simulink model "s01_unicycle"  (R2020a)
settings: Solver=VariableStepAuto  StartTime=0.0  StopTime=20  FixedStep=0.001
InitFcn:
  | clc, close all
  | 
  | run('./s00_config.m')
  | 
  | load('./parameters/ut_obj')
  | load('./parameters/yt_obj')
  | load('./parameters/Kp')
  | load('./parameters/Kr')
  | load('./parameters/Mp')
  | load('./parameters/Mr')
  | 
  | iterSeed = randi(500);
model workspace (MAT data in the model file):
  M : object (value not decoded)
  M_nonlin : object (value not decoded)
  M_tmp : object (value not decoded)
  RHS : object (value not decoded)
  RHS_nonlin : object (value not decoded)
  RHS_tmp : object (value not decoded)
  Tp : object (value not decoded)
  Tp_var = 0
  Tw : object (value not decoded)
  Tw_var = 0
  op_trim3 : handle (value not decoded)
  q1 : object (value not decoded)
  q1_d : object (value not decoded)
  q2 : object (value not decoded)
  q2_d : object (value not decoded)
  q3 : object (value not decoded)
  q3_d : object (value not decoded)
  q4 : object (value not decoded)
  q4_d : object (value not decoded)
  q5 : object (value not decoded)
  q5_d : object (value not decoded)
  z = [0 0 0 0 0 0 0 0 0 0 0 0 ... (100 elements, 10x10)]
values from neighbouring files (symbols this model uses):
  b_disc = 0.01    [s00_config.m]
  Bp = [B_p1 B_p2 B_p3 B_p4]    [s00_config.m]    (also in s00_designLQR.m = double([0; b2; 0; b4]))
  flag_AddPitchBias = 0    [s00_config.m]
  flag_AddRollBias = 0    [s00_config.m]
  flag_UseAccNoise = 1    [s00_config.m]
  flag_useControlDelay = 0    [s00_config.m]
  flag_UseGyroNoise = 1    [s00_config.m]
  flag_UsePitchEst = 1    [s00_config.m]
  flag_UsePivotAcc = 1    [s00_config.m]
  flag_UseRateEst = 1    [s00_config.m]
  flag_UseRollEst = 1    [s00_config.m]
  flag_UseYawEst = 1    [s00_config.m]
  Icx = 0.001746    [s00_config.m]
  Icy = 0.00181    [s00_config.m]
  Icz = 0.001585    [s00_config.m]
  Iwx = 0.000259    [s00_config.m]
  Iwy = 0.000503    [s00_config.m]
  Iwz = 0.000259    [s00_config.m]
  Lc = 0.055    [s00_config.m]
  Lcp = 0.055    [s00_config.m]
  mean_IMUgyro = -0.0065    [s00_config.m]
  pitch_bias = deg2rad(1)    [s00_config.m]
  q1_0 = -deg2rad(36)    [s00_config.m]
  q2_0 = deg2rad(0)    [s00_config.m]
  r = Rw - 0.01    (= 0.043)    [s00_config.m]
  roll_bias = deg2rad(1)    [s00_config.m]
  Rw = 0.053    [s00_config.m]
  stall_torque = 1.6    [s00_config.m]
  Ts = 1/100    (= 0.01)    [s00_config.m]
  variance_IMUacc = 0.0049    [s00_config.m]
  variance_IMUgyro = 6.3956e-04    (= 0.00063956)    [s00_config.m]
  X = (P.')/(P*P.')    [s00_config.m]
  Xp = X(:,1)    [s00_config.m]
undefined symbols (not defined in the file or in its folder): DiscIntNeverNeededParam, sigbuilder_block, Y, Z
libraries: sm_lib x59, aerolibconvert2 x11, nesl_utility x8, eeGeneralControl x2, simulink x1, SignalEditorBlockLib x1
(part 2 of 2)

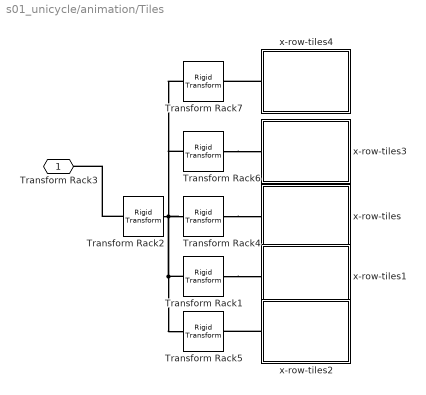
== system s01_unicycle/animation/Tiles ==
  Transform Rack1 : sm_lib/Frames and Transforms/Rigid Transform  TranslationMethod=StandardAxis  TranslationStandardOffset=0.25  TranslationLengthUnit=m  TranslationStandardAxis=-Y  TranslationCartesianOffset=[0 0 0]  TranslationROffset=0  TranslationROffsetUnits=m  TranslationZOffset=0  TranslationZOffsetUnits=m  TranslationThetaOffset=0  TranslationThetaOffsetUnits=deg  RotationMethod=None  RotationAngleUnits=deg  RotationStandardAxis=-X  RotationAngle=90  RotationArbitraryAxis=[0 0 1]  FollAlignAxisA=+X  BaseAlignAxisA=+Y  FollAlignAxisB=+Y  BaseAlignAxisB=+Z  RotationSequenceAxes=FollowerAxes  RotationSequence=XYX  RotationSequenceAngles=[0 0 0]  RotationSequenceAnglesUnits=deg  RotationMatrix=[1 0 0; 0 1 0; 0 0 1]
  Transform Rack2 : sm_lib/Frames and Transforms/Rigid Transform  TranslationMethod=StandardAxis  TranslationStandardOffset=0.001  TranslationLengthUnit=m  TranslationStandardAxis=+Z  TranslationCartesianOffset=[0 0 0]  TranslationROffset=0  TranslationROffsetUnits=m  TranslationZOffset=0  TranslationZOffsetUnits=m  TranslationThetaOffset=0  TranslationThetaOffsetUnits=deg  RotationMethod=None  RotationAngleUnits=deg  RotationStandardAxis=-X  RotationAngle=90  RotationArbitraryAxis=[0 0 1]  FollAlignAxisA=+X  BaseAlignAxisA=+Y  FollAlignAxisB=+Y  BaseAlignAxisB=+Z  RotationSequenceAxes=FollowerAxes  RotationSequence=XYX  RotationSequenceAngles=[0 0 0]  RotationSequenceAnglesUnits=deg  RotationMatrix=[1 0 0; 0 1 0; 0 0 1]
  Transform Rack4 : sm_lib/Frames and Transforms/Rigid Transform  TranslationMethod=StandardAxis  TranslationStandardOffset=0  TranslationLengthUnit=m  TranslationStandardAxis=-Y  TranslationCartesianOffset=[0 0 0]  TranslationROffset=0  TranslationROffsetUnits=m  TranslationZOffset=0  TranslationZOffsetUnits=m  TranslationThetaOffset=0  TranslationThetaOffsetUnits=deg  RotationMethod=None  RotationAngleUnits=deg  RotationStandardAxis=-X  RotationAngle=90  RotationArbitraryAxis=[0 0 1]  FollAlignAxisA=+X  BaseAlignAxisA=+Y  FollAlignAxisB=+Y  BaseAlignAxisB=+Z  RotationSequenceAxes=FollowerAxes  RotationSequence=XYX  RotationSequenceAngles=[0 0 0]  RotationSequenceAnglesUnits=deg  RotationMatrix=[1 0 0; 0 1 0; 0 0 1]
  Transform Rack5 : sm_lib/Frames and Transforms/Rigid Transform  TranslationMethod=StandardAxis  TranslationStandardOffset=0.25  TranslationLengthUnit=m  TranslationStandardAxis=+Y  TranslationCartesianOffset=[0 0 0]  TranslationROffset=0  TranslationROffsetUnits=m  TranslationZOffset=0  TranslationZOffsetUnits=m  TranslationThetaOffset=0  TranslationThetaOffsetUnits=deg  RotationMethod=None  RotationAngleUnits=deg  RotationStandardAxis=-X  RotationAngle=90  RotationArbitraryAxis=[0 0 1]  FollAlignAxisA=+X  BaseAlignAxisA=+Y  FollAlignAxisB=+Y  BaseAlignAxisB=+Z  RotationSequenceAxes=FollowerAxes  RotationSequence=XYX  RotationSequenceAngles=[0 0 0]  RotationSequenceAnglesUnits=deg  RotationMatrix=[1 0 0; 0 1 0; 0 0 1]
  Transform Rack6 : sm_lib/Frames and Transforms/Rigid Transform  TranslationMethod=StandardAxis  TranslationStandardOffset=0.5  TranslationLengthUnit=m  TranslationStandardAxis=-Y  TranslationCartesianOffset=[0 0 0]  TranslationROffset=0  TranslationROffsetUnits=m  TranslationZOffset=0  TranslationZOffsetUnits=m  TranslationThetaOffset=0  TranslationThetaOffsetUnits=deg  RotationMethod=None  RotationAngleUnits=deg  RotationStandardAxis=-X  RotationAngle=90  RotationArbitraryAxis=[0 0 1]  FollAlignAxisA=+X  BaseAlignAxisA=+Y  FollAlignAxisB=+Y  BaseAlignAxisB=+Z  RotationSequenceAxes=FollowerAxes  RotationSequence=XYX  RotationSequenceAngles=[0 0 0]  RotationSequenceAnglesUnits=deg  RotationMatrix=[1 0 0; 0 1 0; 0 0 1]
  Transform Rack7 : sm_lib/Frames and Transforms/Rigid Transform  TranslationMethod=StandardAxis  TranslationStandardOffset=0.5  TranslationLengthUnit=m  TranslationStandardAxis=+Y  TranslationCartesianOffset=[0 0 0]  TranslationROffset=0  TranslationROffsetUnits=m  TranslationZOffset=0  TranslationZOffsetUnits=m  TranslationThetaOffset=0  TranslationThetaOffsetUnits=deg  RotationMethod=None  RotationAngleUnits=deg  RotationStandardAxis=-X  RotationAngle=90  RotationArbitraryAxis=[0 0 1]  FollAlignAxisA=+X  BaseAlignAxisA=+Y  FollAlignAxisB=+Y  BaseAlignAxisB=+Z  RotationSequenceAxes=FollowerAxes  RotationSequence=XYX  RotationSequenceAngles=[0 0 0]  RotationSequenceAnglesUnits=deg  RotationMatrix=[1 0 0; 0 1 0; 0 0 1]
  x-row-tiles : Subsystem
  x-row-tiles1 : Subsystem
  x-row-tiles2 : Subsystem
  x-row-tiles3 : Subsystem
  x-row-tiles4 : Subsystem
  Transform Rack3 : PMIOPort  Side=Left
  connections:
  Transform Rack1/LConn1 -- Transform Rack7/LConn1 -- Transform Rack6/LConn1 -- Transform Rack4/LConn1 -- Transform Rack2/RConn1 -- Transform Rack5/LConn1
  x-row-tiles4/LConn1 -- Transform Rack7/RConn1
  x-row-tiles2/LConn1 -- Transform Rack5/RConn1
  Transform Rack4/RConn1 -- x-row-tiles/LConn1
  Transform Rack1/RConn1 -- x-row-tiles1/LConn1
  Transform Rack2/LConn1 -- Transform Rack3/RConn1
  Transform Rack6/RConn1 -- x-row-tiles3/LConn1

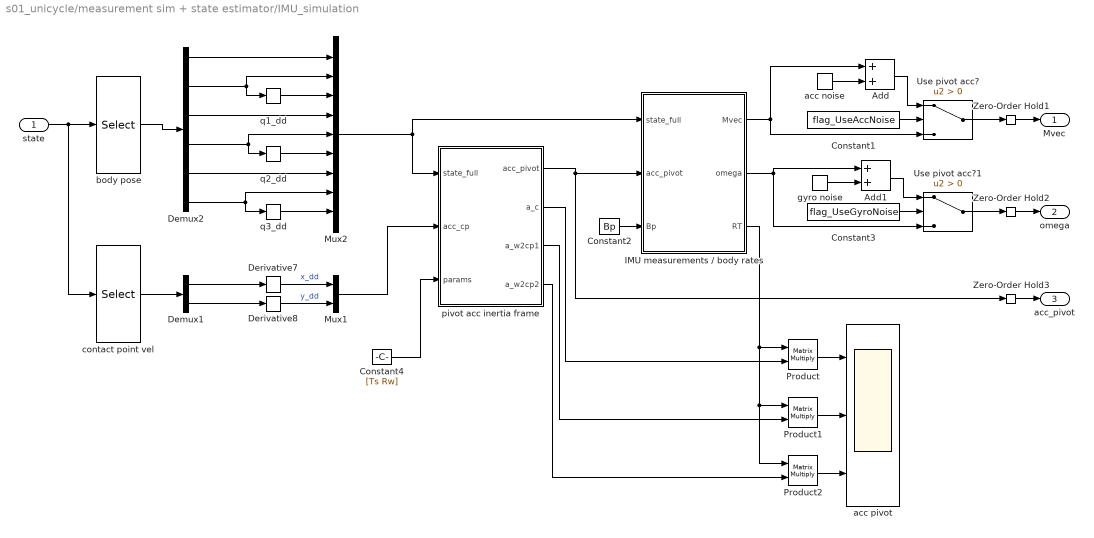
== system s01_unicycle/measurement sim + state estimator/IMU_simulation ==
  state : Inport
  Add : Sum
  Add1 : Sum
  Constant1 : Constant  Value=flag_UseAccNoise
  Constant2 : Constant  Value=Bp
  Constant3 : Constant  Value=flag_UseGyroNoise
  Constant4 : Constant  Value=[Ts Rw]
  Demux1 : Demux  Outputs=2
  Demux2 : Demux  Outputs=6
  Derivative7 : Derivative  CoefficientInTFapproximation=0.00001
  Derivative8 : Derivative  CoefficientInTFapproximation=0.00001
  IMU measurements / body rates : MATLAB Function  TreatAsAtomicUnit=on
  Mux1 : Mux  Inputs=2
  Mux2 : Mux  Inputs=9
  Product : Product  Multiplication=Matrix(*)
  Product1 : Product  Multiplication=Matrix(*)
  Product2 : Product  Multiplication=Matrix(*)
  Use pivot acc? : Switch  Criteria=u2 > Threshold
  Use pivot acc?1 : Switch  Criteria=u2 > Threshold
  Zero-Order Hold1 : ZeroOrderHold  SampleTime=Ts
  Zero-Order Hold2 : ZeroOrderHold  SampleTime=Ts
  Zero-Order Hold3 : ZeroOrderHold  SampleTime=Ts
  acc noise : RandomNumber  Mean=zeros(1,12)  Variance=variance_IMUacc*ones(1,12)  Seed=1:12  SampleTime=Ts
  acc pivot : Scope  NumInputPorts=3
  body pose : Selector  InputPortWidth=14  IndexOptions=Index vector (dialog)  Indices=[1 2 3 4 5 6]  OutputSizes=1
  contact point vel : Selector  InputPortWidth=14  IndexOptions=Index vector (dialog)  Indices=[13, 14]  OutputSizes=1
  gyro noise : RandomNumber  Mean=mean_IMUgyro*[1 1 1]  Variance=(variance_IMUgyro)*[1 1 1]  Seed=[iterSeed+10 iterSeed+11 iterSeed+12]  SampleTime=Ts
  pivot acc inertia frame : MATLAB Function  TreatAsAtomicUnit=on
  q1_dd : Derivative  CoefficientInTFapproximation=0.0000001
  q2_dd : Derivative  CoefficientInTFapproximation=0.000001
  q3_dd : Derivative  CoefficientInTFapproximation=0.000001
  Mvec : Outport
  omega : Outport  Port=2
  acc_pivot : Outport  Port=3
  wires:
  Demux2/2 -> Mux2/2, q1_dd/1
  Mux2/1 -> IMU measurements / body rates/1(state_full), pivot acc inertia frame/1(state_full)
  state/1 -> contact point vel/1, body pose/1
  Demux2/6 -> Mux2/8, q3_dd/1
  Demux1/1 -> Derivative7/1
  gyro noise/1 -> Add1/2
  IMU measurements / body rates/1(Mvec) -> Use pivot acc?/3, Add/1
  Constant2/1 -> IMU measurements / body rates/3(Bp)
  Demux2/4 -> Mux2/5, q2_dd/1
  IMU measurements / body rates/2(omega) -> Use pivot acc?1/3, Add1/1
  q2_dd/1 -> Mux2/6
  q1_dd/1 -> Mux2/3
  contact point vel/1 -> Demux1/1
  Derivative8/1 -> Mux1/2  "y_dd"
  Demux2/5 -> Mux2/7
  Demux2/1 -> Mux2/1
  Mux1/1 -> pivot acc inertia frame/2(acc_cp)
  pivot acc inertia frame/1(acc_pivot) -> Zero-Order Hold3/1, IMU measurements / body rates/2(acc_pivot)
  Derivative7/1 -> Mux1/1  "x_dd"
  body pose/1 -> Demux2/1
  Demux2/3 -> Mux2/4
  Demux1/2 -> Derivative8/1
  acc noise/1 -> Add/2
  q3_dd/1 -> Mux2/9
  Constant4/1 -> pivot acc inertia frame/3(params)
  Zero-Order Hold1/1 -> Mvec/1
  Zero-Order Hold2/1 -> omega/1
  Zero-Order Hold3/1 -> acc_pivot/1
  Use pivot acc?/1 -> Zero-Order Hold1/1
  Add/1 -> Use pivot acc?/1
  Constant1/1 -> Use pivot acc?/2
  Constant3/1 -> Use pivot acc?1/2
  Use pivot acc?1/1 -> Zero-Order Hold2/1
  Add1/1 -> Use pivot acc?1/1
  pivot acc inertia frame/2(a_c) -> Product/2
  pivot acc inertia frame/3(a_w2cp1) -> Product1/2
  pivot acc inertia frame/4(a_w2cp2) -> Product2/2
  IMU measurements / body rates/3(RT) -> Product2/1, Product1/1, Product/1
  Product/1 -> acc pivot/1
  Product2/1 -> acc pivot/3
  Product1/1 -> acc pivot/2

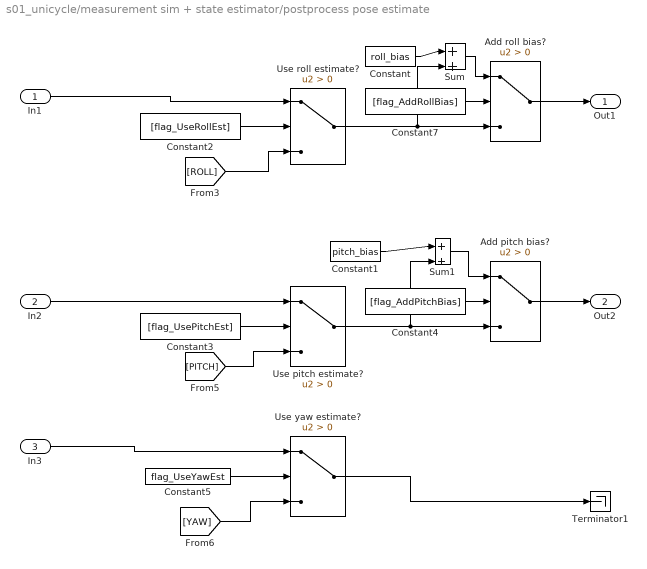
== system s01_unicycle/measurement sim + state estimator/postprocess pose estimate ==
  In1 : Inport
  In2 : Inport  Port=2
  In3 : Inport  Port=3
  Add pitch bias? : Switch  Criteria=u2 > Threshold
  Add roll bias? : Switch  Criteria=u2 > Threshold
  Constant : Constant  Value=roll_bias
  Constant1 : Constant  Value=pitch_bias
  Constant2 : Constant  Value=[flag_UseRollEst]
  Constant3 : Constant  Value=[flag_UsePitchEst]
  Constant4 : Constant  Value=[flag_AddPitchBias]
  Constant5 : Constant  Value=flag_UseYawEst
  Constant7 : Constant  Value=[flag_AddRollBias]
  Sum : Sum  Inputs=|++
  Sum1 : Sum  Inputs=|++
  Terminator1 : Terminator
  Use pitch estimate? : Switch  Criteria=u2 > Threshold
  Use roll estimate? : Switch  Criteria=u2 > Threshold
  Use yaw estimate? : Switch  Criteria=u2 > Threshold
  Out1 : Outport
  Out2 : Outport  Port=2
  wires:
  [ROLL] -> Use roll estimate?/3
  Use yaw estimate?/1 -> Terminator1/1
  Constant7/1 -> Add roll bias?/2
  Constant2/1 -> Use roll estimate?/2
  [YAW] -> Use yaw estimate?/3
  [PITCH] -> Use pitch estimate?/3
  In2/1 -> Use pitch estimate?/1
  Sum/1 -> Add roll bias?/1
  Use roll estimate?/1 -> Sum/2, Add roll bias?/3
  Constant/1 -> Sum/1
  Constant5/1 -> Use yaw estimate?/2
  Constant3/1 -> Use pitch estimate?/2
  In3/1 -> Use yaw estimate?/1
  Add roll bias?/1 -> Out1/1
  In1/1 -> Use roll estimate?/1
  Use pitch estimate?/1 -> Sum1/2, Add pitch bias?/3
  Sum1/1 -> Add pitch bias?/1
  Add pitch bias?/1 -> Out2/1
  Constant4/1 -> Add pitch bias?/2
  Constant1/1 -> Sum1/1

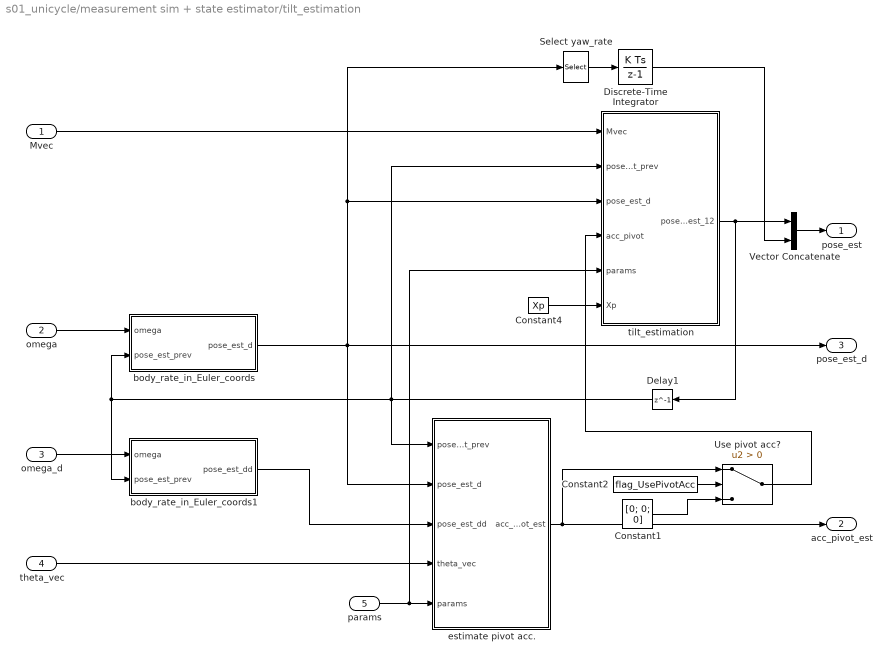
== system s01_unicycle/measurement sim + state estimator/tilt_estimation ==
  Mvec : Inport
  omega : Inport  Port=2
  omega_d : Inport  Port=3
  theta_vec : Inport  Port=4  PortDimensions=3
  params : Inport  Port=5
  Constant1 : Constant  Value="[0;  0; 0]"
  Constant2 : Constant  Value=flag_UsePivotAcc
  Constant4 : Constant  Value=Xp
  Delay1 : Delay  DelayLength=1  InitialCondition=[q1_0; q2_0]  SampleTime=Ts
  Discrete-Time Integrator : DiscreteIntegrator  SampleTime=-1  ICPrevOutput=DiscIntNeverNeededParam  ICPrevScaledInput=DiscIntNeverNeededParam
  Select yaw_rate : Selector  InputPortWidth=3  IndexOptions=Index vector (dialog)  Indices=[3]  OutputSizes=1
  Use pivot acc? : Switch  Criteria=u2 > Threshold
  Vector Concatenate : Concatenate
  body_rate_in_Euler_coords : MATLAB Function  TreatAsAtomicUnit=on
  body_rate_in_Euler_coords1 : MATLAB Function  TreatAsAtomicUnit=on
  estimate pivot acc. : MATLAB Function  TreatAsAtomicUnit=on
  tilt_estimation : MATLAB Function  TreatAsAtomicUnit=on
  pose_est : Outport
  acc_pivot_est : Outport  Port=2
  pose_est_d : Outport  Port=3
  wires:
  estimate pivot acc./1(acc_pivot_est) -> Use pivot acc?/1, acc_pivot_est/1
  Delay1/1 -> estimate pivot acc./1(pose_est_prev), body_rate_in_Euler_coords/2(pose_est_prev), body_rate_in_Euler_coords1/2(pose_est_prev), tilt_estimation/2(pose_est_prev)
  body_rate_in_Euler_coords/1(pose_est_d) -> pose_est_d/1, Select yaw_rate/1, tilt_estimation/3(pose_est_d), estimate pivot acc./2(pose_est_d)
  Select yaw_rate/1 -> Discrete-Time Integrator/1
  omega_d/1 -> body_rate_in_Euler_coords1/1(omega)
  body_rate_in_Euler_coords1/1(pose_est_dd) -> estimate pivot acc./3(pose_est_dd)
  Use pivot acc?/1 -> tilt_estimation/4(acc_pivot)
  omega/1 -> body_rate_in_Euler_coords/1(omega)
  params/1 -> tilt_estimation/5(params), estimate pivot acc./5(params)
  tilt_estimation/1(pose_est_12) -> Vector Concatenate/1, Delay1/1
  Mvec/1 -> tilt_estimation/1(Mvec)
  Vector Concatenate/1 -> pose_est/1
  Constant4/1 -> tilt_estimation/6(Xp)
  Constant1/1 -> Use pivot acc?/3
  Constant2/1 -> Use pivot acc?/2
  Discrete-Time Integrator/1 -> Vector Concatenate/2
  theta_vec/1 -> estimate pivot acc./4(theta_vec)

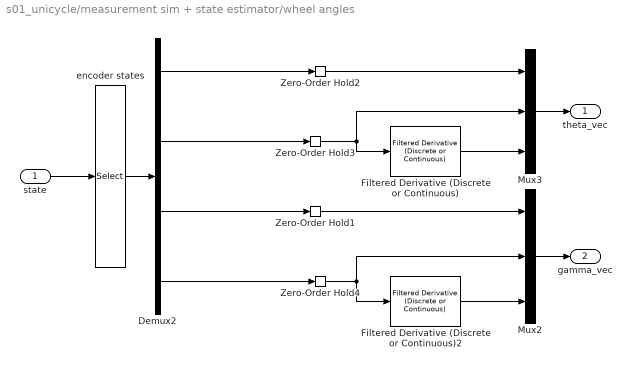
== system s01_unicycle/measurement sim + state estimator/wheel angles ==
  state : Inport
  Demux2 : Demux
  Filtered Derivative (Discrete or Continuous) : eeGeneralControl/Filtered Derivative (Discrete or Continuous)  K=1  T=0.1  B=inf  A=-inf  minRatio=10  init_option=Inherited from block input  x0=0  Ts=-1
      settings: SourceProductBaseCode=PS
  Filtered Derivative (Discrete or Continuous)2 : eeGeneralControl/Filtered Derivative (Discrete or Continuous)  K=1  T=0.1  B=inf  A=-inf  minRatio=10  init_option=Inherited from block input  x0=0  Ts=-1
      settings: SourceProductBaseCode=PS
  Mux2 : Mux  Inputs=3
  Mux3 : Mux  Inputs=3
  Zero-Order Hold{1..4} (4 alike) : ZeroOrderHold  SampleTime=Ts
  encoder states : Selector  InputPortWidth=14  IndexOptions=Index vector (dialog)  Indices=[7, 8, 9, 10]  OutputSizes=1
  theta_vec : Outport
  gamma_vec : Outport  Port=2
  wires:
  Demux2/3 -> Zero-Order Hold1/1
  encoder states/1 -> Demux2/1
  Zero-Order Hold3/1 -> Mux3/2, Filtered Derivative (Discrete or Continuous)/1
  Demux2/2 -> Zero-Order Hold3/1
  Demux2/1 -> Zero-Order Hold2/1
  state/1 -> encoder states/1
  Filtered Derivative (Discrete or Continuous)/1 -> Mux3/3
  Demux2/4 -> Zero-Order Hold4/1
  Zero-Order Hold4/1 -> Mux2/2, Filtered Derivative (Discrete or Continuous)2/1
  Filtered Derivative (Discrete or Continuous)2/1 -> Mux2/3
  Mux3/1 -> theta_vec/1
  Zero-Order Hold1/1 -> Mux2/1
  Mux2/1 -> gamma_vec/1
  Zero-Order Hold2/1 -> Mux3/1

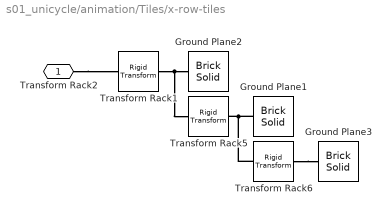
== system s01_unicycle/animation/Tiles/x-row-tiles ==
  Ground Plane1 : sm_lib/Body Elements/Brick Solid  GraphicAmbientColor=[0.15 0.15 0 1.0]  BasedOnType=Density  BrickDimensions=[0.25 0.25 0.001]  BrickDimensionUnits=m  CenterOfMass=[0 0 0]  CenterOfMassUnits=m  GraphicDiffuseColor=[1.0 1.0 1.0]  Density=100  DensityUnits=kg/(m^3)  DoExposeReferenceFrame=on  GraphicEmissiveColor=[0.0 0.0 0.0 1.0]  ExportEntireGeometry=off  SerializedFrames=<Frames/>  MarkerShape=Cube  MarkerSize=10000  GraphicType=FromGeometry  InertiaType=CalculateFromGeometry  Mass=1  MassUnits=kg  MomentsOfInertia=[1 1 1]  MomentsOfInertiaUnits=kg*m^2  GraphicOpacity=1  ProductsOfInertia=[0 0 0]  ProductsOfInertiaUnits=kg*m^2  GraphicShininess=75  GraphicSpecularColor=[0.5 0.5 0.1 1.0]  GraphicVisPropType=SimpleVisualProperties
  Ground Plane2 : sm_lib/Body Elements/Brick Solid  GraphicAmbientColor=[0.15 0.15 0 1.0]  BasedOnType=Density  BrickDimensions=[0.25 0.25 0.001]  BrickDimensionUnits=m  CenterOfMass=[0 0 0]  CenterOfMassUnits=m  GraphicDiffuseColor=[1.0 1.0 1.0]  Density=100  DensityUnits=kg/(m^3)  DoExposeReferenceFrame=on  GraphicEmissiveColor=[0.0 0.0 0.0 1.0]  ExportEntireGeometry=off  SerializedFrames=<Frames/>  MarkerShape=Cube  MarkerSize=10000  GraphicType=FromGeometry  InertiaType=CalculateFromGeometry  Mass=1  MassUnits=kg  MomentsOfInertia=[1 1 1]  MomentsOfInertiaUnits=kg*m^2  GraphicOpacity=1  ProductsOfInertia=[0 0 0]  ProductsOfInertiaUnits=kg*m^2  GraphicShininess=75  GraphicSpecularColor=[0.5 0.5 0.1 1.0]  GraphicVisPropType=SimpleVisualProperties
  Ground Plane3 : sm_lib/Body Elements/Brick Solid  GraphicAmbientColor=[0.15 0.15 0 1.0]  BasedOnType=Density  BrickDimensions=[0.25 0.25 0.001]  BrickDimensionUnits=m  CenterOfMass=[0 0 0]  CenterOfMassUnits=m  GraphicDiffuseColor=[1.0 1.0 1.0]  Density=100  DensityUnits=kg/(m^3)  DoExposeReferenceFrame=on  GraphicEmissiveColor=[0.0 0.0 0.0 1.0]  ExportEntireGeometry=off  SerializedFrames=<Frames/>  MarkerShape=Cube  MarkerSize=10000  GraphicType=FromGeometry  InertiaType=CalculateFromGeometry  Mass=1  MassUnits=kg  MomentsOfInertia=[1 1 1]  MomentsOfInertiaUnits=kg*m^2  GraphicOpacity=1  ProductsOfInertia=[0 0 0]  ProductsOfInertiaUnits=kg*m^2  GraphicShininess=75  GraphicSpecularColor=[0.5 0.5 0.1 1.0]  GraphicVisPropType=SimpleVisualProperties
  Transform Rack1 : sm_lib/Frames and Transforms/Rigid Transform  TranslationMethod=StandardAxis  TranslationStandardOffset=0.625  TranslationLengthUnit=m  TranslationStandardAxis=-X  TranslationCartesianOffset=[0 0 0]  TranslationROffset=0  TranslationROffsetUnits=m  TranslationZOffset=0  TranslationZOffsetUnits=m  TranslationThetaOffset=0  TranslationThetaOffsetUnits=deg  RotationMethod=None  RotationAngleUnits=deg  RotationStandardAxis=-X  RotationAngle=90  RotationArbitraryAxis=[0 0 1]  FollAlignAxisA=+X  BaseAlignAxisA=+Y  FollAlignAxisB=+Y  BaseAlignAxisB=+Z  RotationSequenceAxes=FollowerAxes  RotationSequence=XYX  RotationSequenceAngles=[0 0 0]  RotationSequenceAnglesUnits=deg  RotationMatrix=[1 0 0; 0 1 0; 0 0 1]
  Transform Rack5 : sm_lib/Frames and Transforms/Rigid Transform  TranslationMethod=StandardAxis  TranslationStandardOffset=0.5  TranslationLengthUnit=m  TranslationStandardAxis=+X  TranslationCartesianOffset=[0 0 0]  TranslationROffset=0  TranslationROffsetUnits=m  TranslationZOffset=0  TranslationZOffsetUnits=m  TranslationThetaOffset=0  TranslationThetaOffsetUnits=deg  RotationMethod=None  RotationAngleUnits=deg  RotationStandardAxis=-X  RotationAngle=90  RotationArbitraryAxis=[0 0 1]  FollAlignAxisA=+X  BaseAlignAxisA=+Y  FollAlignAxisB=+Y  BaseAlignAxisB=+Z  RotationSequenceAxes=FollowerAxes  RotationSequence=XYX  RotationSequenceAngles=[0 0 0]  RotationSequenceAnglesUnits=deg  RotationMatrix=[1 0 0; 0 1 0; 0 0 1]
  Transform Rack6 : sm_lib/Frames and Transforms/Rigid Transform  TranslationMethod=StandardAxis  TranslationStandardOffset=0.5  TranslationLengthUnit=m  TranslationStandardAxis=+X  TranslationCartesianOffset=[0 0 0]  TranslationROffset=0  TranslationROffsetUnits=m  TranslationZOffset=0  TranslationZOffsetUnits=m  TranslationThetaOffset=0  TranslationThetaOffsetUnits=deg  RotationMethod=None  RotationAngleUnits=deg  RotationStandardAxis=-X  RotationAngle=90  RotationArbitraryAxis=[0 0 1]  FollAlignAxisA=+X  BaseAlignAxisA=+Y  FollAlignAxisB=+Y  BaseAlignAxisB=+Z  RotationSequenceAxes=FollowerAxes  RotationSequence=XYX  RotationSequenceAngles=[0 0 0]  RotationSequenceAnglesUnits=deg  RotationMatrix=[1 0 0; 0 1 0; 0 0 1]
  Transform Rack2 : PMIOPort  Side=Left
  connections:
  Transform Rack1/RConn1 -- Transform Rack5/LConn1 -- Ground Plane2/RConn1
  Transform Rack6/RConn1 -- Ground Plane3/RConn1
  Ground Plane1/RConn1 -- Transform Rack6/LConn1 -- Transform Rack5/RConn1
  Transform Rack2/RConn1 -- Transform Rack1/LConn1

== system s01_unicycle/animation/Tiles/x-row-tiles1 ==
  Ground Plane1 : sm_lib/Body Elements/Brick Solid  GraphicAmbientColor=[0.15 0.15 0 1.0]  BasedOnType=Density  BrickDimensions=[0.25 0.25 0.001]  BrickDimensionUnits=m  CenterOfMass=[0 0 0]  CenterOfMassUnits=m  GraphicDiffuseColor=[1.0 1.0 1.0]  Density=100  DensityUnits=kg/(m^3)  DoExposeReferenceFrame=on  GraphicEmissiveColor=[0.0 0.0 0.0 1.0]  ExportEntireGeometry=off  SerializedFrames=<Frames/>  MarkerShape=Cube  MarkerSize=10000  GraphicType=FromGeometry  InertiaType=CalculateFromGeometry  Mass=1  MassUnits=kg  MomentsOfInertia=[1 1 1]  MomentsOfInertiaUnits=kg*m^2  GraphicOpacity=1  ProductsOfInertia=[0 0 0]  ProductsOfInertiaUnits=kg*m^2  GraphicShininess=75  GraphicSpecularColor=[0.5 0.5 0.1 1.0]  GraphicVisPropType=SimpleVisualProperties
  Ground Plane2 : sm_lib/Body Elements/Brick Solid  GraphicAmbientColor=[0.15 0.15 0 1.0]  BasedOnType=Density  BrickDimensions=[0.25 0.25 0.001]  BrickDimensionUnits=m  CenterOfMass=[0 0 0]  CenterOfMassUnits=m  GraphicDiffuseColor=[1.0 1.0 1.0]  Density=100  DensityUnits=kg/(m^3)  DoExposeReferenceFrame=on  GraphicEmissiveColor=[0.0 0.0 0.0 1.0]  ExportEntireGeometry=off  SerializedFrames=<Frames/>  MarkerShape=Cube  MarkerSize=10000  GraphicType=FromGeometry  InertiaType=CalculateFromGeometry  Mass=1  MassUnits=kg  MomentsOfInertia=[1 1 1]  MomentsOfInertiaUnits=kg*m^2  GraphicOpacity=1  ProductsOfInertia=[0 0 0]  ProductsOfInertiaUnits=kg*m^2  GraphicShininess=75  GraphicSpecularColor=[0.5 0.5 0.1 1.0]  GraphicVisPropType=SimpleVisualProperties
  Transform Rack1 : sm_lib/Frames and Transforms/Rigid Transform  TranslationMethod=StandardAxis  TranslationStandardOffset=0.375  TranslationLengthUnit=m  TranslationStandardAxis=-X  TranslationCartesianOffset=[0 0 0]  TranslationROffset=0  TranslationROffsetUnits=m  TranslationZOffset=0  TranslationZOffsetUnits=m  TranslationThetaOffset=0  TranslationThetaOffsetUnits=deg  RotationMethod=None  RotationAngleUnits=deg  RotationStandardAxis=-X  RotationAngle=90  RotationArbitraryAxis=[0 0 1]  FollAlignAxisA=+X  BaseAlignAxisA=+Y  FollAlignAxisB=+Y  BaseAlignAxisB=+Z  RotationSequenceAxes=FollowerAxes  RotationSequence=XYX  RotationSequenceAngles=[0 0 0]  RotationSequenceAnglesUnits=deg  RotationMatrix=[1 0 0; 0 1 0; 0 0 1]
  Transform Rack5 : sm_lib/Frames and Transforms/Rigid Transform  TranslationMethod=StandardAxis  TranslationStandardOffset=0.5  TranslationLengthUnit=m  TranslationStandardAxis=+X  TranslationCartesianOffset=[0 0 0]  TranslationROffset=0  TranslationROffsetUnits=m  TranslationZOffset=0  TranslationZOffsetUnits=m  TranslationThetaOffset=0  TranslationThetaOffsetUnits=deg  RotationMethod=None  RotationAngleUnits=deg  RotationStandardAxis=-X  RotationAngle=90  RotationArbitraryAxis=[0 0 1]  FollAlignAxisA=+X  BaseAlignAxisA=+Y  FollAlignAxisB=+Y  BaseAlignAxisB=+Z  RotationSequenceAxes=FollowerAxes  RotationSequence=XYX  RotationSequenceAngles=[0 0 0]  RotationSequenceAnglesUnits=deg  RotationMatrix=[1 0 0; 0 1 0; 0 0 1]
  Transform Rack2 : PMIOPort  Side=Left
  connections:
  Transform Rack1/RConn1 -- Ground Plane2/RConn1 -- Transform Rack5/LConn1
  Ground Plane1/RConn1 -- Transform Rack5/RConn1
  Transform Rack2/RConn1 -- Transform Rack1/LConn1

== system s01_unicycle/animation/Tiles/x-row-tiles2 ==
  Ground Plane1 : sm_lib/Body Elements/Brick Solid  GraphicAmbientColor=[0.15 0.15 0 1.0]  BasedOnType=Density  BrickDimensions=[0.25 0.25 0.001]  BrickDimensionUnits=m  CenterOfMass=[0 0 0]  CenterOfMassUnits=m  GraphicDiffuseColor=[1.0 1.0 1.0]  Density=100  DensityUnits=kg/(m^3)  DoExposeReferenceFrame=on  GraphicEmissiveColor=[0.0 0.0 0.0 1.0]  ExportEntireGeometry=off  SerializedFrames=<Frames/>  MarkerShape=Cube  MarkerSize=10000  GraphicType=FromGeometry  InertiaType=CalculateFromGeometry  Mass=1  MassUnits=kg  MomentsOfInertia=[1 1 1]  MomentsOfInertiaUnits=kg*m^2  GraphicOpacity=1  ProductsOfInertia=[0 0 0]  ProductsOfInertiaUnits=kg*m^2  GraphicShininess=75  GraphicSpecularColor=[0.5 0.5 0.1 1.0]  GraphicVisPropType=SimpleVisualProperties
  Ground Plane2 : sm_lib/Body Elements/Brick Solid  GraphicAmbientColor=[0.15 0.15 0 1.0]  BasedOnType=Density  BrickDimensions=[0.25 0.25 0.001]  BrickDimensionUnits=m  CenterOfMass=[0 0 0]  CenterOfMassUnits=m  GraphicDiffuseColor=[1.0 1.0 1.0]  Density=100  DensityUnits=kg/(m^3)  DoExposeReferenceFrame=on  GraphicEmissiveColor=[0.0 0.0 0.0 1.0]  ExportEntireGeometry=off  SerializedFrames=<Frames/>  MarkerShape=Cube  MarkerSize=10000  GraphicType=FromGeometry  InertiaType=CalculateFromGeometry  Mass=1  MassUnits=kg  MomentsOfInertia=[1 1 1]  MomentsOfInertiaUnits=kg*m^2  GraphicOpacity=1  ProductsOfInertia=[0 0 0]  ProductsOfInertiaUnits=kg*m^2  GraphicShininess=75  GraphicSpecularColor=[0.5 0.5 0.1 1.0]  GraphicVisPropType=SimpleVisualProperties
  Transform Rack1 : sm_lib/Frames and Transforms/Rigid Transform  TranslationMethod=StandardAxis  TranslationStandardOffset=0.375  TranslationLengthUnit=m  TranslationStandardAxis=-X  TranslationCartesianOffset=[0 0 0]  TranslationROffset=0  TranslationROffsetUnits=m  TranslationZOffset=0  TranslationZOffsetUnits=m  TranslationThetaOffset=0  TranslationThetaOffsetUnits=deg  RotationMethod=None  RotationAngleUnits=deg  RotationStandardAxis=-X  RotationAngle=90  RotationArbitraryAxis=[0 0 1]  FollAlignAxisA=+X  BaseAlignAxisA=+Y  FollAlignAxisB=+Y  BaseAlignAxisB=+Z  RotationSequenceAxes=FollowerAxes  RotationSequence=XYX  RotationSequenceAngles=[0 0 0]  RotationSequenceAnglesUnits=deg  RotationMatrix=[1 0 0; 0 1 0; 0 0 1]
  Transform Rack5 : sm_lib/Frames and Transforms/Rigid Transform  TranslationMethod=StandardAxis  TranslationStandardOffset=0.5  TranslationLengthUnit=m  TranslationStandardAxis=+X  TranslationCartesianOffset=[0 0 0]  TranslationROffset=0  TranslationROffsetUnits=m  TranslationZOffset=0  TranslationZOffsetUnits=m  TranslationThetaOffset=0  TranslationThetaOffsetUnits=deg  RotationMethod=None  RotationAngleUnits=deg  RotationStandardAxis=-X  RotationAngle=90  RotationArbitraryAxis=[0 0 1]  FollAlignAxisA=+X  BaseAlignAxisA=+Y  FollAlignAxisB=+Y  BaseAlignAxisB=+Z  RotationSequenceAxes=FollowerAxes  RotationSequence=XYX  RotationSequenceAngles=[0 0 0]  RotationSequenceAnglesUnits=deg  RotationMatrix=[1 0 0; 0 1 0; 0 0 1]
  Transform Rack2 : PMIOPort  Side=Left
  connections:
  Transform Rack1/RConn1 -- Ground Plane2/RConn1 -- Transform Rack5/LConn1
  Ground Plane1/RConn1 -- Transform Rack5/RConn1
  Transform Rack2/RConn1 -- Transform Rack1/LConn1

== system s01_unicycle/animation/Tiles/x-row-tiles3 ==
  Ground Plane1 : sm_lib/Body Elements/Brick Solid  GraphicAmbientColor=[0.15 0.15 0 1.0]  BasedOnType=Density  BrickDimensions=[0.25 0.25 0.001]  BrickDimensionUnits=m  CenterOfMass=[0 0 0]  CenterOfMassUnits=m  GraphicDiffuseColor=[1.0 1.0 1.0]  Density=100  DensityUnits=kg/(m^3)  DoExposeReferenceFrame=on  GraphicEmissiveColor=[0.0 0.0 0.0 1.0]  ExportEntireGeometry=off  SerializedFrames=<Frames/>  MarkerShape=Cube  MarkerSize=10000  GraphicType=FromGeometry  InertiaType=CalculateFromGeometry  Mass=1  MassUnits=kg  MomentsOfInertia=[1 1 1]  MomentsOfInertiaUnits=kg*m^2  GraphicOpacity=1  ProductsOfInertia=[0 0 0]  ProductsOfInertiaUnits=kg*m^2  GraphicShininess=75  GraphicSpecularColor=[0.5 0.5 0.1 1.0]  GraphicVisPropType=SimpleVisualProperties
  Ground Plane2 : sm_lib/Body Elements/Brick Solid  GraphicAmbientColor=[0.15 0.15 0 1.0]  BasedOnType=Density  BrickDimensions=[0.25 0.25 0.001]  BrickDimensionUnits=m  CenterOfMass=[0 0 0]  CenterOfMassUnits=m  GraphicDiffuseColor=[1.0 1.0 1.0]  Density=100  DensityUnits=kg/(m^3)  DoExposeReferenceFrame=on  GraphicEmissiveColor=[0.0 0.0 0.0 1.0]  ExportEntireGeometry=off  SerializedFrames=<Frames/>  MarkerShape=Cube  MarkerSize=10000  GraphicType=FromGeometry  InertiaType=CalculateFromGeometry  Mass=1  MassUnits=kg  MomentsOfInertia=[1 1 1]  MomentsOfInertiaUnits=kg*m^2  GraphicOpacity=1  ProductsOfInertia=[0 0 0]  ProductsOfInertiaUnits=kg*m^2  GraphicShininess=75  GraphicSpecularColor=[0.5 0.5 0.1 1.0]  GraphicVisPropType=SimpleVisualProperties
  Ground Plane3 : sm_lib/Body Elements/Brick Solid  GraphicAmbientColor=[0.15 0.15 0 1.0]  BasedOnType=Density  BrickDimensions=[0.25 0.25 0.001]  BrickDimensionUnits=m  CenterOfMass=[0 0 0]  CenterOfMassUnits=m  GraphicDiffuseColor=[1.0 1.0 1.0]  Density=100  DensityUnits=kg/(m^3)  DoExposeReferenceFrame=on  GraphicEmissiveColor=[0.0 0.0 0.0 1.0]  ExportEntireGeometry=off  SerializedFrames=<Frames/>  MarkerShape=Cube  MarkerSize=10000  GraphicType=FromGeometry  InertiaType=CalculateFromGeometry  Mass=1  MassUnits=kg  MomentsOfInertia=[1 1 1]  MomentsOfInertiaUnits=kg*m^2  GraphicOpacity=1  ProductsOfInertia=[0 0 0]  ProductsOfInertiaUnits=kg*m^2  GraphicShininess=75  GraphicSpecularColor=[0.5 0.5 0.1 1.0]  GraphicVisPropType=SimpleVisualProperties
  Transform Rack1 : sm_lib/Frames and Transforms/Rigid Transform  TranslationMethod=StandardAxis  TranslationStandardOffset=0.625  TranslationLengthUnit=m  TranslationStandardAxis=-X  TranslationCartesianOffset=[0 0 0]  TranslationROffset=0  TranslationROffsetUnits=m  TranslationZOffset=0  TranslationZOffsetUnits=m  TranslationThetaOffset=0  TranslationThetaOffsetUnits=deg  RotationMethod=None  RotationAngleUnits=deg  RotationStandardAxis=-X  RotationAngle=90  RotationArbitraryAxis=[0 0 1]  FollAlignAxisA=+X  BaseAlignAxisA=+Y  FollAlignAxisB=+Y  BaseAlignAxisB=+Z  RotationSequenceAxes=FollowerAxes  RotationSequence=XYX  RotationSequenceAngles=[0 0 0]  RotationSequenceAnglesUnits=deg  RotationMatrix=[1 0 0; 0 1 0; 0 0 1]
  Transform Rack5 : sm_lib/Frames and Transforms/Rigid Transform  TranslationMethod=StandardAxis  TranslationStandardOffset=0.5  TranslationLengthUnit=m  TranslationStandardAxis=+X  TranslationCartesianOffset=[0 0 0]  TranslationROffset=0  TranslationROffsetUnits=m  TranslationZOffset=0  TranslationZOffsetUnits=m  TranslationThetaOffset=0  TranslationThetaOffsetUnits=deg  RotationMethod=None  RotationAngleUnits=deg  RotationStandardAxis=-X  RotationAngle=90  RotationArbitraryAxis=[0 0 1]  FollAlignAxisA=+X  BaseAlignAxisA=+Y  FollAlignAxisB=+Y  BaseAlignAxisB=+Z  RotationSequenceAxes=FollowerAxes  RotationSequence=XYX  RotationSequenceAngles=[0 0 0]  RotationSequenceAnglesUnits=deg  RotationMatrix=[1 0 0; 0 1 0; 0 0 1]
  Transform Rack6 : sm_lib/Frames and Transforms/Rigid Transform  TranslationMethod=StandardAxis  TranslationStandardOffset=0.5  TranslationLengthUnit=m  TranslationStandardAxis=+X  TranslationCartesianOffset=[0 0 0]  TranslationROffset=0  TranslationROffsetUnits=m  TranslationZOffset=0  TranslationZOffsetUnits=m  TranslationThetaOffset=0  TranslationThetaOffsetUnits=deg  RotationMethod=None  RotationAngleUnits=deg  RotationStandardAxis=-X  RotationAngle=90  RotationArbitraryAxis=[0 0 1]  FollAlignAxisA=+X  BaseAlignAxisA=+Y  FollAlignAxisB=+Y  BaseAlignAxisB=+Z  RotationSequenceAxes=FollowerAxes  RotationSequence=XYX  RotationSequenceAngles=[0 0 0]  RotationSequenceAnglesUnits=deg  RotationMatrix=[1 0 0; 0 1 0; 0 0 1]
  Transform Rack2 : PMIOPort  Side=Left
  connections:
  Transform Rack1/RConn1 -- Ground Plane2/RConn1 -- Transform Rack5/LConn1
  Transform Rack6/RConn1 -- Ground Plane3/RConn1
  Transform Rack5/RConn1 -- Ground Plane1/RConn1 -- Transform Rack6/LConn1
  Transform Rack2/RConn1 -- Transform Rack1/LConn1

== system s01_unicycle/animation/Tiles/x-row-tiles4 ==
  Ground Plane1 : sm_lib/Body Elements/Brick Solid  GraphicAmbientColor=[0.15 0.15 0 1.0]  BasedOnType=Density  BrickDimensions=[0.25 0.25 0.001]  BrickDimensionUnits=m  CenterOfMass=[0 0 0]  CenterOfMassUnits=m  GraphicDiffuseColor=[1.0 1.0 1.0]  Density=100  DensityUnits=kg/(m^3)  DoExposeReferenceFrame=on  GraphicEmissiveColor=[0.0 0.0 0.0 1.0]  ExportEntireGeometry=off  SerializedFrames=<Frames/>  MarkerShape=Cube  MarkerSize=10000  GraphicType=FromGeometry  InertiaType=CalculateFromGeometry  Mass=1  MassUnits=kg  MomentsOfInertia=[1 1 1]  MomentsOfInertiaUnits=kg*m^2  GraphicOpacity=1  ProductsOfInertia=[0 0 0]  ProductsOfInertiaUnits=kg*m^2  GraphicShininess=75  GraphicSpecularColor=[0.5 0.5 0.1 1.0]  GraphicVisPropType=SimpleVisualProperties
  Ground Plane2 : sm_lib/Body Elements/Brick Solid  GraphicAmbientColor=[0.15 0.15 0 1.0]  BasedOnType=Density  BrickDimensions=[0.25 0.25 0.001]  BrickDimensionUnits=m  CenterOfMass=[0 0 0]  CenterOfMassUnits=m  GraphicDiffuseColor=[1.0 1.0 1.0]  Density=100  DensityUnits=kg/(m^3)  DoExposeReferenceFrame=on  GraphicEmissiveColor=[0.0 0.0 0.0 1.0]  ExportEntireGeometry=off  SerializedFrames=<Frames/>  MarkerShape=Cube  MarkerSize=10000  GraphicType=FromGeometry  InertiaType=CalculateFromGeometry  Mass=1  MassUnits=kg  MomentsOfInertia=[1 1 1]  MomentsOfInertiaUnits=kg*m^2  GraphicOpacity=1  ProductsOfInertia=[0 0 0]  ProductsOfInertiaUnits=kg*m^2  GraphicShininess=75  GraphicSpecularColor=[0.5 0.5 0.1 1.0]  GraphicVisPropType=SimpleVisualProperties
  Ground Plane3 : sm_lib/Body Elements/Brick Solid  GraphicAmbientColor=[0.15 0.15 0 1.0]  BasedOnType=Density  BrickDimensions=[0.25 0.25 0.001]  BrickDimensionUnits=m  CenterOfMass=[0 0 0]  CenterOfMassUnits=m  GraphicDiffuseColor=[1.0 1.0 1.0]  Density=100  DensityUnits=kg/(m^3)  DoExposeReferenceFrame=on  GraphicEmissiveColor=[0.0 0.0 0.0 1.0]  ExportEntireGeometry=off  SerializedFrames=<Frames/>  MarkerShape=Cube  MarkerSize=10000  GraphicType=FromGeometry  InertiaType=CalculateFromGeometry  Mass=1  MassUnits=kg  MomentsOfInertia=[1 1 1]  MomentsOfInertiaUnits=kg*m^2  GraphicOpacity=1  ProductsOfInertia=[0 0 0]  ProductsOfInertiaUnits=kg*m^2  GraphicShininess=75  GraphicSpecularColor=[0.5 0.5 0.1 1.0]  GraphicVisPropType=SimpleVisualProperties
  Transform Rack1 : sm_lib/Frames and Transforms/Rigid Transform  TranslationMethod=StandardAxis  TranslationStandardOffset=0.625  TranslationLengthUnit=m  TranslationStandardAxis=-X  TranslationCartesianOffset=[0 0 0]  TranslationROffset=0  TranslationROffsetUnits=m  TranslationZOffset=0  TranslationZOffsetUnits=m  TranslationThetaOffset=0  TranslationThetaOffsetUnits=deg  RotationMethod=None  RotationAngleUnits=deg  RotationStandardAxis=-X  RotationAngle=90  RotationArbitraryAxis=[0 0 1]  FollAlignAxisA=+X  BaseAlignAxisA=+Y  FollAlignAxisB=+Y  BaseAlignAxisB=+Z  RotationSequenceAxes=FollowerAxes  RotationSequence=XYX  RotationSequenceAngles=[0 0 0]  RotationSequenceAnglesUnits=deg  RotationMatrix=[1 0 0; 0 1 0; 0 0 1]
  Transform Rack5 : sm_lib/Frames and Transforms/Rigid Transform  TranslationMethod=StandardAxis  TranslationStandardOffset=0.5  TranslationLengthUnit=m  TranslationStandardAxis=+X  TranslationCartesianOffset=[0 0 0]  TranslationROffset=0  TranslationROffsetUnits=m  TranslationZOffset=0  TranslationZOffsetUnits=m  TranslationThetaOffset=0  TranslationThetaOffsetUnits=deg  RotationMethod=None  RotationAngleUnits=deg  RotationStandardAxis=-X  RotationAngle=90  RotationArbitraryAxis=[0 0 1]  FollAlignAxisA=+X  BaseAlignAxisA=+Y  FollAlignAxisB=+Y  BaseAlignAxisB=+Z  RotationSequenceAxes=FollowerAxes  RotationSequence=XYX  RotationSequenceAngles=[0 0 0]  RotationSequenceAnglesUnits=deg  RotationMatrix=[1 0 0; 0 1 0; 0 0 1]
  Transform Rack6 : sm_lib/Frames and Transforms/Rigid Transform  TranslationMethod=StandardAxis  TranslationStandardOffset=0.5  TranslationLengthUnit=m  TranslationStandardAxis=+X  TranslationCartesianOffset=[0 0 0]  TranslationROffset=0  TranslationROffsetUnits=m  TranslationZOffset=0  TranslationZOffsetUnits=m  TranslationThetaOffset=0  TranslationThetaOffsetUnits=deg  RotationMethod=None  RotationAngleUnits=deg  RotationStandardAxis=-X  RotationAngle=90  RotationArbitraryAxis=[0 0 1]  FollAlignAxisA=+X  BaseAlignAxisA=+Y  FollAlignAxisB=+Y  BaseAlignAxisB=+Z  RotationSequenceAxes=FollowerAxes  RotationSequence=XYX  RotationSequenceAngles=[0 0 0]  RotationSequenceAnglesUnits=deg  RotationMatrix=[1 0 0; 0 1 0; 0 0 1]
  Transform Rack2 : PMIOPort  Side=Left
  connections:
  Transform Rack1/RConn1 -- Ground Plane2/RConn1 -- Transform Rack5/LConn1
  Transform Rack6/RConn1 -- Ground Plane3/RConn1
  Transform Rack5/RConn1 -- Ground Plane1/RConn1 -- Transform Rack6/LConn1
  Transform Rack2/RConn1 -- Transform Rack1/LConn1

== matlab function s01_unicycle/Tw_forward ==
  data: q2 input; u_w output
function u_w = fcn(q2)
    u_w = (-0.055 * 0.75 * 9.81 * sin(q2) -  (2*0.055) * 0.3 * 9.81 * sin(q2));
end

== matlab function s01_unicycle/MATLAB Function ==
  data: rate input; y output; torque input
function y = saturate_torque(rate, torque)

    if abs(rate) > 282
       y = 0;
    else
       y = torque;
    end
end

== matlab function s01_unicycle/measurement sim + state estimator/IMU_simulation/IMU measurements // body rates ==
  data: state_full input; acc_pivot input; Mvec output; omega output; Bp input; RT output
function [Mvec, omega, RT] = fcn(state_full, acc_pivot, Bp)
% Computes acceleration measurements of all four IMUS in their respective
% Coord-sys, Note that the transform from global-coord. to COG-coord. is
% via YAW -> ROLL -> PITCH

q1 = state_full(1);  % Roll "alpha" (Euler angle)
q1_d = state_full(2);
q1_dd = state_full(3);
q2 = state_full(4);  % Pitch "beta" (Euler angle)
q2_d = state_full(5);
q2_dd = state_full(6);
q3 = state_full(7);  % Yaw "delta" (Euler angle)
q3_d = state_full(8);
q3_dd = state_full(9);

Ry = [cos(q2) 0 sin(q2);0 1 0;-sin(q2) 0 cos(q2)];  % From c to w2
Rx = [1 0 0;0 cos(q1) -sin(q1);0 sin(q1) cos(q1)];  % From w2 to cp
Rz = [cos(q3) -sin(q3) 0;sin(q3) cos(q3) 0;0 0 1];  % From cp to g
R = Rz*Rx*Ry; % from body to inertia (yaw roll pitch)
RT = R.'; % from inertía to body (yaw roll pitch)

% Transform the euler rate/acc. to body angular rate/acc.
omega = Ry.' * Rx.' * [0.0; 0.0; q3_d] + Ry.'*[q1_d; 0.0; 0.0] + [0.0; q2_d; 0.0];
omega_d = Ry.' * Rx.' * [0.0; 0.0; q3_dd] + Ry.'*[q1_dd; 0.0; 0.0] + [0.0; q2_dd; 0.0];  

omega_skew = [[0 -omega(3), omega(2)]; [omega(3), 0, -omega(1)];[-omega(2), omega(1), 0]];
omega_skew_d = [[0 -omega_d(3), omega_d(2)]; [omega_d(3) 0 -omega_d(1)];[-omega_d(2) omega_d(1) 0]];
B_omega = omega_skew*omega_skew + omega_skew_d;

% IMU position vectors Bp in body-fixed frame (frame origin is  at pivot point)
% Note that acc_pivot and g are invariant to Rz.T
g = 9.81;
B_g = RT*[0;0;g]; 

Mvec = [RT*acc_pivot + B_g + B_omega*Bp(:,1);
        RT*acc_pivot + B_g + B_omega*Bp(:,2);
        RT*acc_pivot + B_g + B_omega*Bp(:,3);
        RT*acc_pivot + B_g + B_omega*Bp(:,4)];
end

== matlab function s01_unicycle/measurement sim + state estimator/IMU_simulation/pivot acc inertia frame ==
  data: state_full input; acc_cp input; params input; acc_pivot output; a_c output; a_w2cp1 output; a_w2cp2 output
function [acc_pivot, a_c, a_w2cp1, a_w2cp2]  = fcn(state_full, acc_cp, params)
% Computes acceleration measurements of all four IMUS in their respective
% Coord-sys, Note that the transform from global-coord. to COG-coord. is
% via YAW -> ROLL -> PITCH
Rw = params(2);

q1 = state_full(1);  % Roll "alpha" (Euler angle)
q1_d = state_full(2);
q1_dd = state_full(3);

q3 = state_full(7);  % Yaw "delta" (Euler angle)
q3_d = state_full(8);
q3_dd = state_full(9);

% Compute pivot point acc. in global frame 
% (a_w2cp1: velocity dependend)
a_w2cp_x1 = cos(q3)*(2*Rw*cos(q1)*q3_d*q1_d) - sin(q3)*(Rw*sin(q1)*q3_d^2+Rw*sin(q1)*q1_d^2);
a_w2cp_y1 = sin(q3)*(2*Rw*cos(q1)*q3_d*q1_d) + cos(q3)*(Rw*sin(q1)*q3_d^2+Rw*sin(q1)*q1_d^2);
a_w2cp_z1 = -Rw*cos(q1)*q1_d^2;
a_w2cp1 = [a_w2cp_x1; a_w2cp_y1; a_w2cp_z1];
% (a_w2cp2: acceleration dependend)
a_w2cp_x2 = Rw*cos(q3)*sin(q1)*q3_dd + Rw*sin(q3)*cos(q1)*q1_dd;
a_w2cp_y2 = Rw*sin(q3)*sin(q1)*q3_dd - Rw*cos(q3)*cos(q1)*q1_dd;
a_w2cp_z2 = -Rw*sin(q1)*q1_dd;
a_w2cp2 = [a_w2cp_x2; a_w2cp_y2; a_w2cp_z2];

a_c = [acc_cp(1); acc_cp(2); 0];

acc_pivot = a_c + a_w2cp1 + a_w2cp2; % Note that the acc. of the piv point consists of a_w2cp and a_cpg
end

== matlab function s01_unicycle/measurement sim + state estimator/tilt_estimation/body_rate_in_Euler_coords ==
  data: omega input; pose_est_prev input; pose_est_d output
function pose_est_d   = fcn(omega, pose_est_prev)
% Compute euler rates and angular acc from noisy body rates

q1 = pose_est_prev(1);
q2 = pose_est_prev(2);

body2euler = [[cos(q2), 0, sin(q2)];
              [ 0, 1, 0];
              [ -cos(q1)*sin(q2), sin(q1), cos(q1)*cos(q2)]];
   
pose_est_d = body2euler * omega;
end

== matlab function s01_unicycle/measurement sim + state estimator/tilt_estimation_old ==
  data: params input; Xp input; Mvec input; pose_est output; omega input; omega_d input; pose_est_prev input; theta_vec input
function pose_est  = fcn(params, Xp, Mvec, omega, omega_d, pose_est_prev, theta_vec)
Ts = params(1);
Rw = params(2);

q1 = pose_est_prev(1);
q2 = pose_est_prev(2);

% Rotation matrices for computing pivot point acc.
Ry = [cos(q2) 0 sin(q2); 0 1 0; -sin(q2) 0 cos(q2)]; % From c to w2
Rx = [1 0 0; 0 cos(q1) -sin(q1); 0 sin(q1) cos(q1)]; % From w2 to cp

% Compute euler rates and angular acc from noisy body rates
body2euler = [[cos(q2), 0, sin(q2)];
              [ 0, 1, 0];
              [ -cos(q1)*sin(q2), sin(q1), cos(q1)*cos(q2)]];
   
q_d = body2euler * omega;
q_dd = body2euler * omega_d;

q1_d = q_d(1);
q2_d = q_d(2);
q3_d = q_d(3);
q4_d = theta_vec(2);

q1_dd = q_dd(1);
%q2_dd = q_dd(2);
q3_dd = q_dd(3);
q4_dd = theta_vec(3);

% Contact point acc in global frame already transformed by Rz.' 
a_cp = [Rw*q4_dd; Rw*q4_d*q3_d; 0]; % Note that cos(q3) is gone due to Rz.'

% Compute contact to pivot point acc. in global frame already transformed by Rz.' 
% (a_w2cp1: velocity dependend, a_w2cp2: acceleration dependend)

a_w2cp_x1 = 2*Rw*cos(q1)*q3_d*q1_d;
a_w2cp_y1 = Rw*sin(q1)*q3_d^2+Rw*sin(q1)*q1_d^2;
a_w2cp_z1 = -Rw*cos(q1)*q1_d^2;
a_w2cp1 = [a_w2cp_x1; a_w2cp_y1; a_w2cp_z1];

a_w2cp_x2 = Rw*sin(q1)*q3_dd;
a_w2cp_y2 = - Rw*cos(q1)*q1_dd;
a_w2cp_z2 = -Rw*sin(q1)*q1_dd;
a_w2cp2 = [a_w2cp_x2; a_w2cp_y2; a_w2cp_z2];

% Compute pivot point acceleration in body fixed frame
acc_pivot = Ry.'*Rx.'*(a_cp + a_w2cp1 + a_w2cp2); % Note that the acc. of the piv point consists of a_w2cp and a_cp
%acc_pivot = [0; 0; 0];


M = reshape(Mvec-[acc_pivot; acc_pivot; acc_pivot; acc_pivot], [3 length(Mvec)/3]);

% Estimate of gravity vector in body frame
B_gest = M*Xp;

% Fusing the acc. est with gyro est.
k = 0.05; % Fusion parameter
pose_est = [k*atan(B_gest(2)/sqrt(B_gest(1)^2+B_gest(3)^2)) + (1-k)*(q1 + q1_d*Ts);
            k*atan(-B_gest(1)/B_gest(3)) + (1-k)*(q2 + q2_d*Ts)];
end

== matlab function s01_unicycle/measurement sim + state estimator/tilt_estimation/estimate pivot acc. ==
  data: pose_est_prev input; pose_est_d input; pose_est_dd input; theta_vec input; params input; acc_pivot_est output
function acc_pivot_est  = fcn(pose_est_prev, pose_est_d, pose_est_dd, theta_vec, params)
Rw = params(2);

q1 = pose_est_prev(1);
q2 = pose_est_prev(2);

q1_d = pose_est_d(1);
q3_d = pose_est_d(3);
q4_d = theta_vec(2);

q1_dd = pose_est_dd(1);
q3_dd = pose_est_dd(3);
q4_dd = theta_vec(3);

% Rotation matrices for computing pivot point acc.
Ry = [cos(q2) 0 sin(q2); 0 1 0; -sin(q2) 0 cos(q2)]; % From c to w2
Rx = [1 0 0; 0 cos(q1) -sin(q1); 0 sin(q1) cos(q1)]; % From w2 to cp

% Contact point acc in global frame already transformed by Rz.' 
a_cp = [Rw*q4_dd; Rw*q4_d*q3_d; 0]; % Note that cos(q3) is gone due to Rz.'

% Compute contact to pivot point acc. in global frame already transformed by Rz.' 
% (a_w2cp1: velocity dependend, a_w2cp2: acceleration dependend)
a_w2cp_x1 = 2*Rw*cos(q1)*q3_d*q1_d;
a_w2cp_y1 = Rw*sin(q1)*q3_d^2+Rw*sin(q1)*q1_d^2;
a_w2cp_z1 = -Rw*cos(q1)*q1_d^2;
a_w2cp1 = [a_w2cp_x1; a_w2cp_y1; a_w2cp_z1];

a_w2cp_x2 = Rw*sin(q1)*q3_dd;
a_w2cp_y2 = - Rw*cos(q1)*q1_dd;
a_w2cp_z2 = -Rw*sin(q1)*q1_dd;
a_w2cp2 = [a_w2cp_x2; a_w2cp_y2; a_w2cp_z2];

% Compute pivot point acceleration in body fixed frame
acc_pivot_est = Ry.'*Rx.'*(a_cp + a_w2cp1 + a_w2cp2); % Note that the acc. of the piv point consists of a_w2cp and a_cp
end

== matlab function s01_unicycle/measurement sim + state estimator/tilt_estimation/tilt_estimation ==
  data: Mvec input; pose_est_prev input; pose_est_d input; acc_pivot input; params input; pose_est_12 output; Xp input
function pose_est_12  = fcn(Mvec, pose_est_prev, pose_est_d, acc_pivot, params, Xp)
Ts = params(1);

q1 = pose_est_prev(1);
q2 = pose_est_prev(2);
q1_d = pose_est_d(1);
q2_d = pose_est_d(2);

% IMU positions with respect to body frame (origin at pivot point)
M = reshape(Mvec-[acc_pivot; acc_pivot; acc_pivot; acc_pivot], [3 length(Mvec)/3]);

% Estimate of gravity vector in body frame
B_gest = M*Xp;

% Fusing the acc. est with gyro est.
k = 0.05; % Fusion parameter
pose_est_12 = [k*atan(B_gest(2)/sqrt(B_gest(1)^2+B_gest(3)^2)) + (1-k)*(q1 + q1_d*Ts);
            k*atan(-B_gest(1)/B_gest(3)) + (1-k)*(q2 + q2_d*Ts)];
end

== matlab function s01_unicycle/measurement sim + state estimator/tilt_estimation/body_rate_in_Euler_coords1 ==
  data: omega input; pose_est_prev input; pose_est_dd output
function pose_est_dd   = fcn(omega, pose_est_prev)
% Compute euler rates and angular acc from noisy body rates

q1 = pose_est_prev(1);
q2 = pose_est_prev(2);

body2euler = [[cos(q2), 0, sin(q2)];
              [ 0, 1, 0];
              [ -cos(q1)*sin(q2), sin(q1), cos(q1)*cos(q2)]];
   
pose_est_dd = body2euler * omega;
end
